simulink model "engine"  (R2025b)
settings: Solver=VariableStepAuto  StartTime=0.0  StopTime=10.0  RelTol=1e-3
undefined symbols (not defined in the file): car
settings Model: Creator=andre  LastModifiedBy=miche

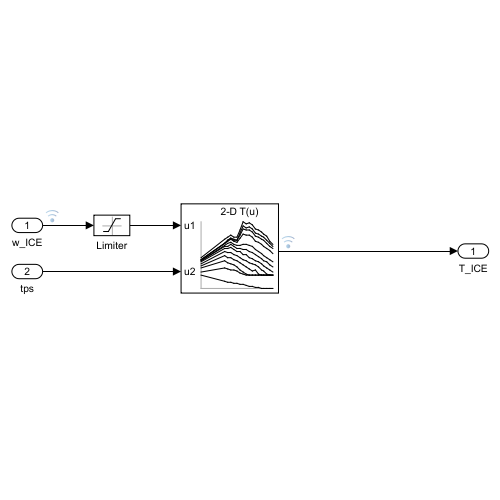
[thumbnail: Simulink's stored preview of the top-level diagram]
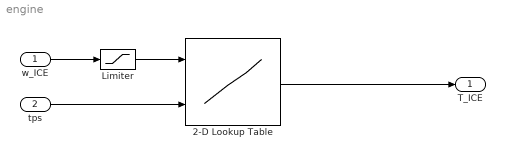
== system engine ==
  w_ICE : Inport
  tps : Inport  Port=2
  2-D Lookup Table : Lookup_n-D  BreakpointsForDimension1=[0;4000;4500;5000;5500;6000;6500;7000;7500;8000;8500;9000;9500;10000;10500;11000;11500;12000]  BreakpointsForDimension2=[0;0.20000000000000001;0.25;0.29999999999999999;0.34999999999999998;0.40000000000000002;0.45000000000000001;0.5;0.59999999999999998;0.69999999999999996;0.80000000000000004;1]  Table=car.engine.lut  InternalRulePriority=Speed  RndMeth=Simplest
      settings: InputPortMap=u0,u1
  Limiter : Saturate  UpperLimit=12500  LowerLimit=4000
  T_ICE : Outport
  wires:
  w_ICE/1 -> Limiter/1
  Limiter/1 -> 2-D Lookup Table/1
  2-D Lookup Table/1 -> T_ICE/1
  tps/1 -> 2-D Lookup Table/2
